simulink model "chap4_1sim"  (R2016a)
settings: Solver=ode45  StartTime=0.0  StopTime=20.0  RelTol=1e-3
settings Model: Creator=zhanghankui  LastModifiedBy=zhanghankui

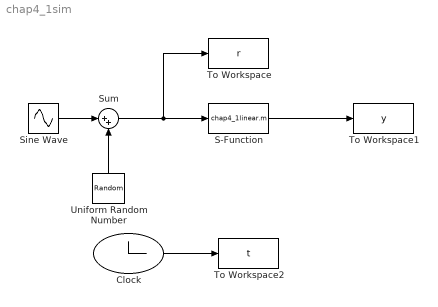
== system chap4_1sim ==
  Clock : Clock
  S-Function : S-Function  FunctionName=chap4_1linear.m  SFunctionDeploymentMode=off  EnableBusSupport=off
  Sine Wave : Sin  SampleTime=0
  Sum : Sum  Inputs=|++
  To Workspace : ToWorkspace  VariableName=r  SaveFormat=Timeseries  SampleTime=-1
  To Workspace1 : ToWorkspace  VariableName=y  SaveFormat=Timeseries  SampleTime=-1
  To Workspace2 : ToWorkspace  VariableName=t  SaveFormat=Timeseries  SampleTime=-1
  Uniform Random Number : UniformRandomNumber  Minimum=0  Maximum=0.05  SampleTime=0.001
  wires:
  Sine Wave/1 -> Sum/1
  Uniform Random Number/1 -> Sum/2
  Sum/1 -> To Workspace/1, S-Function/1
  S-Function/1 -> To Workspace1/1
  Clock/1 -> To Workspace2/1
